simulink library "Actuation_Lib"  (R2026a)
settings: Solver=ode45  EnableMultiTasking=on
undefined symbols (not defined in the file): Mini_Golf_Param, X, Y, Z
libraries: nesl_utility x22, sm_lib x12, Golf_Components_Lib x2, $bdroot x1
Description:
  | Copyright 2015-2026 The MathWorks, Inc.
settings Model: Creator=smiller  LastModifiedBy=smiller
settings DataIOCC: SignalLoggingSaveFormat=ModelDataLogs
settings DebuggingCC: UnderspecifiedInitializationDetection=Classic  PregeneratedLibrarySubsystemCodeDiagnostic=none
settings HardwareCC: ProdHWDeviceType=32-bit Generic

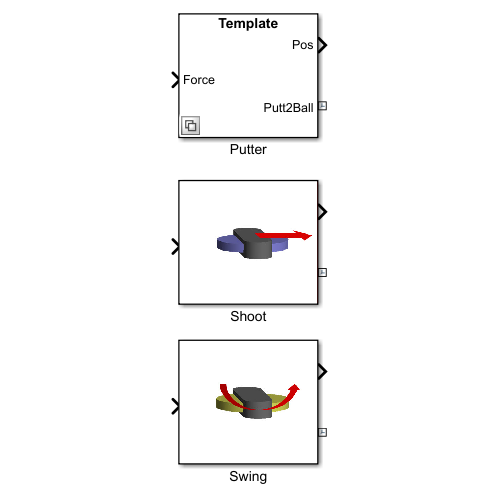
[thumbnail: Simulink's stored preview of the top-level diagram]
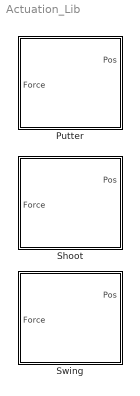
== system Actuation_Lib ==
  Putter : Subsystem  BlockChoice=Shoot
      settings: TemplateBlock=self  MemberBlocks=Shoot,Swing
  Shoot : Subsystem
      mask Display:
      | image(imread('Putter_Shoot_IMAGE.jpg'));
      | %port_label('input',1,'Force');
      | %port_label('output',1,'Pos');
      | %port_label('RConn',1,'Putt2Ball');
  Swing : Subsystem
      mask Display:
      | image(imread('Putter_Swing_IMAGE.jpg'));
      | %port_label('input',1,'Force');
      | %port_label('output',1,'Pos');
      | %port_label('RConn',1,'Putt2Ball');

== system Actuation_Lib/Putter ==
  Force : Inport
  Shoot : $bdroot/Shoot  SystemSampleTime=-1  VariantActivationTime=update diagram  EmptyChoice=off  PassThrough=off  PassThroughVariantControl=(default)  EmptyChoiceVariantControl=(default)  AllowFlexibleInterface=on  Latency=0  AutoFrameSizeCalculation=off
  Putt2Ball : PMIOPort  Side=Right
  Pos : Outport  VectorParamsAs1DForOutWhenUnconnected=off
  wires:
  Force/1 -> Shoot/1
  Shoot/1 -> Pos/1
  connections:
  Shoot/RConn1 -- Putt2Ball/RConn1

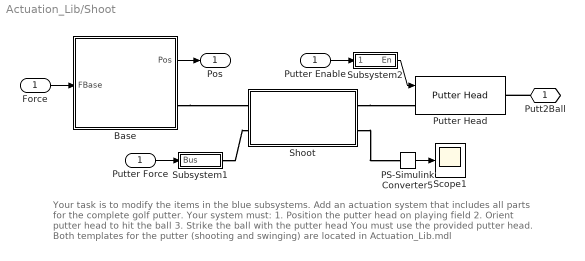
== system Actuation_Lib/Shoot ==
  note: Your task is to modify the items in the blue subsystems.
      | Add an actuation system that includes all parts for the complete golf putter.
      | Your system must:
      | 1. Position the putter head on playing field
      | 2. Orient putter head to hit the ball
      | 3. Strike the ball with the putter head
      |
      | You must use the provided putter head.
      | Both templates for the putter (shooting and swinging) are located in Actuation_Lib.mdl
  Force : Inport
  Base : Subsystem
      mask Display:
      | image(imread('Base_Shoot_IMAGE.jpg'));
      | port_label('input',1,'FBase');
      | port_label('output',1,'Pos');
      | port_label('RConn',1,'CG');
  PS-Simulink Converter5 : nesl_utility/PS-Simulink Converter  PhysicalDomain=network_engine_domain  SubClassName=ps_output  LeftPortType=input  RightPortType=output  PseudoPeriodic=off  Frequencies=[]  VectorFormat=1-D array  Unit=1  AffineConversion=off
  Putter Enable : InportShadow
  Putter Force : InportShadow
  Putter Head : Golf_Components_Lib/Putter Head  length=Mini_Golf_Param.Putter.Length  height=Mini_Golf_Param.Putter.Height  width=Mini_Golf_Param.Putter.Width  ball_radius=Mini_Golf_Param.Ball.Radius  contact_k=Mini_Golf_Param.Wall.Stiffness  contact_b=Mini_Golf_Param.Wall.Damping  low_pass_filt_const=Mini_Golf_Param.Wall.Low_Pass_Filt_Const
  Scope1 : Scope
      settings: DataLoggingVariableName=ScopeData7
  Shoot : Subsystem
      mask Display:
      | image(imread('Shoot_IMAGE.jpg'));
      | port_label('LConn',1,'Actuator');
      | port_label('RConn',1,'Handle');
      | port_label('LConn',2,'Fz');
      | port_label('RConn',2,'p');
  Subsystem1 : Subsystem
  Subsystem2 : Subsystem
  Putt2Ball : PMIOPort  Side=Right
  Pos : Outport  VectorParamsAs1DForOutWhenUnconnected=off
  wires:
  Base/1(Pos) -> Pos/1
  Force/1 -> Base/1(FBase)
  Putter Force/1 -> Subsystem1/1(Bus)
  PS-Simulink Converter5/1 -> Scope1/1
  Putter Enable/1 -> Subsystem2/1(Bus)
  Subsystem2/1(En) -> Putter Head/1
  connections:
  Base/RConn1 -- Shoot/LConn1
  Subsystem1/RConn1 -- Shoot/LConn2
  Shoot/RConn2 -- PS-Simulink Converter5/LConn1
  Putt2Ball/RConn1 -- Putter Head/RConn1
  Shoot/RConn1 -- Putter Head/LConn1

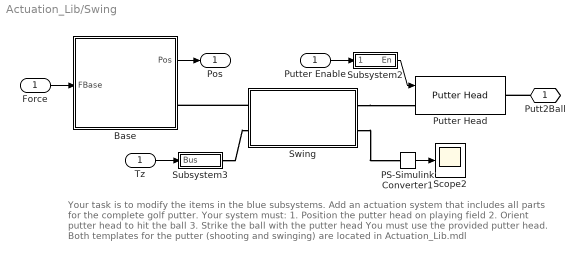
== system Actuation_Lib/Swing ==
  note: Your task is to modify the items in the blue subsystems.
      | Add an actuation system that includes all parts for the complete golf putter.
      | Your system must:
      | 1. Position the putter head on playing field
      | 2. Orient putter head to hit the ball
      | 3. Strike the ball with the putter head
      |
      | You must use the provided putter head.
      | Both templates for the putter (shooting and swinging) are located in Actuation_Lib.mdl
  Force : Inport
  Base : Subsystem
      mask Display:
      | image(imread('Base_Swing_IMAGE.jpg'));
      | port_label('input',1,'FBase');
      | port_label('output',1,'Pos');
      | port_label('RConn',1,'CG');
  PS-Simulink Converter1 : nesl_utility/PS-Simulink Converter  PhysicalDomain=network_engine_domain  SubClassName=ps_output  LeftPortType=input  RightPortType=output  PseudoPeriodic=off  Frequencies=[]  VectorFormat=1-D array  Unit=1  AffineConversion=off
  Putter Enable : InportShadow
  Putter Head : Golf_Components_Lib/Putter Head  length=Mini_Golf_Param.Putter.Length  height=Mini_Golf_Param.Putter.Height  width=Mini_Golf_Param.Putter.Width  ball_radius=Mini_Golf_Param.Ball.Radius  contact_k=Mini_Golf_Param.Wall.Stiffness  contact_b=Mini_Golf_Param.Wall.Damping  low_pass_filt_const=Mini_Golf_Param.Wall.Low_Pass_Filt_Const
  Scope2 : Scope
  Subsystem2 : Subsystem
  Subsystem3 : Subsystem
  Swing : Subsystem
      mask Display:
      | image(imread('Swing_IMAGE.jpg'));
      | port_label('LConn',1,'Actuator');
      | port_label('RConn',1,'Handle');
      | port_label('LConn',2,'Tz');
      | port_label('RConn',2,'p');
  Tz : InportShadow
  Putt2Ball : PMIOPort  Side=Right
  Pos : Outport  VectorParamsAs1DForOutWhenUnconnected=off
  wires:
  Base/1(Pos) -> Pos/1
  Force/1 -> Base/1(FBase)
  Putter Enable/1 -> Subsystem2/1(Bus)
  Subsystem2/1(En) -> Putter Head/1
  Tz/1 -> Subsystem3/1(Bus)
  PS-Simulink Converter1/1 -> Scope2/1
  connections:
  Putt2Ball/RConn1 -- Putter Head/RConn1
  Swing/RConn2 -- PS-Simulink Converter1/LConn1
  Subsystem3/RConn1 -- Swing/LConn2
  Swing/LConn1 -- Base/RConn1
  Swing/RConn1 -- Putter Head/LConn1

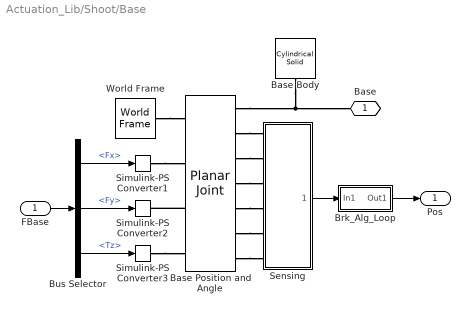
== system Actuation_Lib/Shoot/Base ==
  FBase : Inport
  Base Body : sm_lib/Body Elements/Cylindrical Solid  CylinderRadius=Mini_Golf_Param.Putter.Length*0.5  CylinderRadiusUnits=m  CylinderLength=Mini_Golf_Param.Putter.Height*0.5  CylinderLengthUnits=m  ExportEntireGeometry=off  InertiaType=CalculateFromGeometry  BasedOnType=Mass  Density=1000  DensityUnits=kg/(m^3)  Mass=Mini_Golf_Param.Actuator.Mass  MassUnits=kg  CenterOfMass=[0 0 0]  CenterOfMassUnits=m  MomentsOfInertia=[1 1 1]  MomentsOfInertiaUnits=kg*m^2  ProductsOfInertia=[0 0 0]  ProductsOfInertiaUnits=kg*m^2  GraphicType=FromGeometry  MarkerShape=Sphere  MarkerSize=10  GraphicVisPropType=SimpleVisualProperties  GraphicDiffuseColor=[0.6 0.6 1.0]  GraphicOpacity=1.0  GraphicSpecularColor=[0.5 0.5 0.5 1.0]  GraphicAmbientColor=[0.15 0.15 0.15 1.0]  GraphicEmissiveColor=[0.0 0.0 0.0 1.0]  GraphicShininess=75  DoExposeReferenceFrame=on  SerializedFrames=<Frames/>
  Base Position and Angle : sm_lib/Joints/Planar Joint  JointMode=Normal  CompositeWrenchDir=FollowerOnBase  CompositeWrenchFrame=BaseFrame  SenseConstraintForce=off  SenseConstraintTorque=off  SenseTotalForce=off  SenseTotalTorque=off  PxPositionTargetSpecify=off  PxPositionTargetPriority=High  PxPositionTargetValue=0  PxPositionTargetValueUnits=m  PxVelocityTargetSpecify=off  PxVelocityTargetPriority=High  PxVelocityTargetValue=0  PxVelocityTargetValueUnits=m/s  PxEquilibriumPosition=0  PxEquilibriumPositionUnits=m  PxSpringStiffness=0  PxSpringStiffnessUnits=N/m  PxDampingCoefficient=Mini_Golf_Param.Actuator.Damping_x  PxDampingCoefficientUnits=N/(m/s)  PxLowerLimitSpecify=off  PxLowerLimitBound=-1  PxLowerLimitBoundUnits=m  PxLowerLimitStiffness=1e6  PxLowerLimitStiffnessUnits=N/m  PxLowerLimitDamping=1e3  PxLowerLimitDampingUnits=N/(m/s)  PxLowerLimitTransitionRegionWidth=1e-4  PxLowerLimitTransitionRegionWidthUnits=m  PxUpperLimitSpecify=off  PxUpperLimitBound=1  PxUpperLimitBoundUnits=m  PxUpperLimitStiffness=1e6  PxUpperLimitStiffnessUnits=N/m  PxUpperLimitDamping=1e3  PxUpperLimitDampingUnits=N/(m/s)  PxUpperLimitTransitionRegionWidth=1e-4  PxUpperLimitTransitionRegionWidthUnits=m  PxTorqueActuationMode=InputTorque  PxMotionActuationMode=ComputedMotion  PxSensePosition=on  PxSenseVelocity=on  PxSenseAcceleration=off  PxSenseTorqueForce=off  PxSenseLowerLimitTorqueForce=off  PxSenseUpperLimitTorqueForce=off  PyPositionTargetSpecify=off  PyPositionTargetPriority=High  PyPositionTargetValue=0  PyPositionTargetValueUnits=m  PyVelocityTargetSpecify=off  PyVelocityTargetPriority=High  PyVelocityTargetValue=0  PyVelocityTargetValueUnits=m/s  PyEquilibriumPosition=0  PyEquilibriumPositionUnits=m  PySpringStiffness=0  PySpringStiffnessUnits=N/m  PyDampingCoefficient=Mini_Golf_Param.Actuator.Damping_y  PyDampingCoefficientUnits=N/(m/s)  PyLowerLimitSpecify=off  PyLowerLimitBound=-1  PyLowerLimitBoundUnits=m  PyLowerLimitStiffness=1e6  PyLowerLimitStiffnessUnits=N/m  PyLowerLimitDamping=1e3  PyLowerLimitDampingUnits=N/(m/s)  PyLowerLimitTransitionRegionWidth=1e-4  PyLowerLimitTransitionRegionWidthUnits=m  PyUpperLimitSpecify=off  PyUpperLimitBound=1  PyUpperLimitBoundUnits=m  PyUpperLimitStiffness=1e6  PyUpperLimitStiffnessUnits=N/m  PyUpperLimitDamping=1e3  PyUpperLimitDampingUnits=N/(m/s)  PyUpperLimitTransitionRegionWidth=1e-4  PyUpperLimitTransitionRegionWidthUnits=m  PyTorqueActuationMode=InputTorque  PyMotionActuationMode=ComputedMotion  PySensePosition=on  PySenseVelocity=on  PySenseAcceleration=off  PySenseTorqueForce=off  PySenseLowerLimitTorqueForce=off  PySenseUpperLimitTorqueForce=off  RzPositionTargetSpecify=off  RzPositionTargetPriority=High  RzPositionTargetValue=0  RzPositionTargetValueUnits=rad  RzVelocityTargetSpecify=off  RzVelocityTargetPriority=High  RzVelocityTargetValue=0  RzVelocityTargetValueUnits=rad/s  RzEquilibriumPosition=0  RzEquilibriumPositionUnits=rad  RzSpringStiffness=0  RzSpringStiffnessUnits=N*m/rad  RzDampingCoefficient=Mini_Golf_Param.Actuator.Damping_az  RzDampingCoefficientUnits=N*m/(rad/s)  RzLowerLimitSpecify=off  RzLowerLimitBound=-90  RzLowerLimitBoundUnits=deg  RzLowerLimitStiffness=1e4  RzLowerLimitStiffnessUnits=N*m/deg  RzLowerLimitDamping=10  RzLowerLimitDampingUnits=N*m/(deg/s)  RzLowerLimitTransitionRegionWidth=0.1  RzLowerLimitTransitionRegionWidthUnits=deg  RzUpperLimitSpecify=off  RzUpperLimitBound=90  RzUpperLimitBoundUnits=deg  RzUpperLimitStiffness=1e4  RzUpperLimitStiffnessUnits=N*m/deg  RzUpperLimitDamping=10  RzUpperLimitDampingUnits=N*m/(deg/s)  RzUpperLimitTransitionRegionWidth=0.1  RzUpperLimitTransitionRegionWidthUnits=deg  RzTorqueActuationMode=InputTorque  RzMotionActuationMode=ComputedMotion  RzSensePosition=on  RzSenseVelocity=on  RzSenseAcceleration=off  RzSenseTorqueForce=off  RzSenseLowerLimitTorqueForce=off  RzSenseUpperLimitTorqueForce=off
  Brk_Alg_Loop : Subsystem  mask(First-order lag supporting vector signals){b=Mini_Golf_Param.Actuator.Low_Pass_Filter_Constant, x_initial=0}
      mask prompts: b "Filter time constant"; x_initial "Initial output"
      mask help: Models a lag of the form 1/(b*s+1) where s is the Laplace operator.
  Bus Selector : BusSelector  OutputSignals=Fx,Fy,Tz
  Sensing : Subsystem
  Simulink-PS Converter1 : nesl_utility/Simulink-PS Converter  PhysicalDomain=network_engine_domain  SubClassName=ps_input  LeftPortType=input  RightPortType=output  PseudoPeriodic=off  Frequencies=[]  NoiseDistribution=none  NoiseParameters=[]  Unit=1  AffineConversion=off  FilteringAndDerivatives=zero  SimscapeFilterOrder=1  InputFilterTimeConstant=0.005  UdotUserProvided=0
  Simulink-PS Converter2 : nesl_utility/Simulink-PS Converter  PhysicalDomain=network_engine_domain  SubClassName=ps_input  LeftPortType=input  RightPortType=output  PseudoPeriodic=off  Frequencies=[]  NoiseDistribution=none  NoiseParameters=[]  Unit=1  AffineConversion=off  FilteringAndDerivatives=zero  SimscapeFilterOrder=1  InputFilterTimeConstant=0.005  UdotUserProvided=0
  Simulink-PS Converter3 : nesl_utility/Simulink-PS Converter  PhysicalDomain=network_engine_domain  SubClassName=ps_input  LeftPortType=input  RightPortType=output  PseudoPeriodic=off  Frequencies=[]  NoiseDistribution=none  NoiseParameters=[]  Unit=1  AffineConversion=off  FilteringAndDerivatives=zero  SimscapeFilterOrder=1  InputFilterTimeConstant=0.005  UdotUserProvided=0
  World Frame : sm_lib/Frames and Transforms/World Frame
  Base : PMIOPort  Side=Right
  Pos : Outport  VectorParamsAs1DForOutWhenUnconnected=off
  wires:
  FBase/1 -> Bus Selector/1
  Brk_Alg_Loop/1(Out1) -> Pos/1
  Sensing/1(pos_ang_sig) -> Brk_Alg_Loop/1(In1)
  Bus Selector/1 -> Simulink-PS Converter1/1  "<Fx>"
  Bus Selector/2 -> Simulink-PS Converter2/1  "<Fy>"
  Bus Selector/3 -> Simulink-PS Converter3/1  "<Tz>"
  connections:
  Base Position and Angle/RConn7 -- Sensing/LConn6
  Base Position and Angle/RConn6 -- Sensing/LConn5
  Base Position and Angle/RConn5 -- Sensing/LConn4
  Base Position and Angle/RConn4 -- Sensing/LConn3
  Base Position and Angle/RConn3 -- Sensing/LConn2
  Base Position and Angle/RConn2 -- Sensing/LConn1
  Simulink-PS Converter3/RConn1 -- Base Position and Angle/LConn4
  Base Position and Angle/LConn3 -- Simulink-PS Converter2/RConn1
  Simulink-PS Converter1/RConn1 -- Base Position and Angle/LConn2
  World Frame/RConn1 -- Base Position and Angle/LConn1
  Base Body/RConn1 -- Base Position and Angle/RConn1 -- Base/RConn1

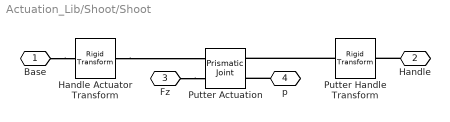
== system Actuation_Lib/Shoot/Shoot ==
  Handle Actuator Transform : sm_lib/Frames and Transforms/Rigid Transform  RotationMethod=StandardAxis  FollAlignAxisA=+X  BaseAlignAxisA=+Y  FollAlignAxisB=+Y  BaseAlignAxisB=+Z  RotationStandardAxis=+Y  RotationAngle=90  RotationAngleUnits=deg  RotationArbitraryAxis=[0 0 1]  RotationSequenceAxes=FollowerAxes  RotationSequence=XYX  RotationSequenceAngles=[0 0 0]  RotationSequenceAnglesUnits=deg  RotationMatrix=[1 0 0; 0 1 0; 0 0 1]  Quaternion=[1 0 0 0]  TranslationMethod=None  TranslationCartesianOffset=[0 0 0]  TranslationCartesianOffsetUnits=m  TranslationStandardAxis=+Z  TranslationStandardOffset=0  TranslationStandardOffsetUnits=m  TranslationROffset=0  TranslationROffsetUnits=m  TranslationThetaOffset=0  TranslationThetaOffsetUnits=deg  TranslationZOffset=0  TranslationZOffsetUnits=m
  Putter Actuation : sm_lib/Joints/Prismatic Joint  JointMode=Normal  CompositeWrenchDir=FollowerOnBase  CompositeWrenchFrame=BaseFrame  SenseConstraintForce=off  SenseConstraintTorque=off  SenseTotalForce=off  SenseTotalTorque=off  PositionTargetSpecify=off  PositionTargetPriority=High  PositionTargetValue=0  PositionTargetValueUnits=m  VelocityTargetSpecify=off  VelocityTargetPriority=High  VelocityTargetValue=0  VelocityTargetValueUnits=m/s  EquilibriumPosition=0  EquilibriumPositionUnits=m  SpringStiffness=Mini_Golf_Param.Actuator.Putter_Spring_k  SpringStiffnessUnits=N/m  DampingCoefficient=Mini_Golf_Param.Actuator.Putter_Damper_b  DampingCoefficientUnits=N/(m/s)  LowerLimitSpecify=off  LowerLimitBound=-1  LowerLimitBoundUnits=m  LowerLimitStiffness=1e6  LowerLimitStiffnessUnits=N/m  LowerLimitDamping=1e3  LowerLimitDampingUnits=N/(m/s)  LowerLimitTransitionRegionWidth=1e-4  LowerLimitTransitionRegionWidthUnits=m  UpperLimitSpecify=off  UpperLimitBound=1  UpperLimitBoundUnits=m  UpperLimitStiffness=1e6  UpperLimitStiffnessUnits=N/m  UpperLimitDamping=1e3  UpperLimitDampingUnits=N/(m/s)  UpperLimitTransitionRegionWidth=1e-4  UpperLimitTransitionRegionWidthUnits=m  TorqueActuationMode=InputTorque  MotionActuationMode=ComputedMotion  SensePosition=on  SenseVelocity=off  SenseAcceleration=off  SenseTorqueForce=off  SenseLowerLimitTorqueForce=off  SenseUpperLimitTorqueForce=off
  Putter Handle Transform : sm_lib/Frames and Transforms/Rigid Transform  RotationMethod=StandardAxis  FollAlignAxisA=+X  BaseAlignAxisA=+Y  FollAlignAxisB=+Y  BaseAlignAxisB=+Z  RotationStandardAxis=+Y  RotationAngle=-90  RotationAngleUnits=deg  RotationArbitraryAxis=[0 0 1]  RotationSequenceAxes=FollowerAxes  RotationSequence=XYX  RotationSequenceAngles=[0 0 0]  RotationSequenceAnglesUnits=deg  RotationMatrix=[1 0 0; 0 1 0; 0 0 1]  Quaternion=[1 0 0 0]  TranslationMethod=None  TranslationCartesianOffset=[0 0 0]  TranslationCartesianOffsetUnits=m  TranslationStandardAxis=+Z  TranslationStandardOffset=0  TranslationStandardOffsetUnits=m  TranslationROffset=0  TranslationROffsetUnits=m  TranslationThetaOffset=0  TranslationThetaOffsetUnits=deg  TranslationZOffset=0  TranslationZOffsetUnits=m
  Base : PMIOPort  Side=Left
  Handle : PMIOPort  Port=2  Side=Right
  Fz : PMIOPort  Port=3  Side=Left
  p : PMIOPort  Port=4  Side=Right
  connections:
  p/RConn1 -- Putter Actuation/RConn2
  Fz/RConn1 -- Putter Actuation/LConn2
  Handle/RConn1 -- Putter Handle Transform/RConn1
  Base/RConn1 -- Handle Actuator Transform/LConn1
  Putter Handle Transform/LConn1 -- Putter Actuation/RConn1
  Handle Actuator Transform/RConn1 -- Putter Actuation/LConn1

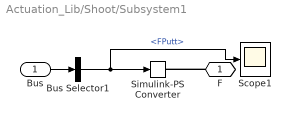
== system Actuation_Lib/Shoot/Subsystem1 ==
  Bus : Inport
  Bus Selector1 : BusSelector  OutputSignals=FPutt
  Scope1 : Scope
      settings: DataLoggingVariableName=ScopeData11
  Simulink-PS Converter : nesl_utility/Simulink-PS Converter  PhysicalDomain=network_engine_domain  SubClassName=ps_input  LeftPortType=input  RightPortType=output  PseudoPeriodic=off  Frequencies=[]  NoiseDistribution=none  NoiseParameters=[]  Unit=1  AffineConversion=off  FilteringAndDerivatives=zero  SimscapeFilterOrder=1  InputFilterTimeConstant=0.005  UdotUserProvided=0
  F : PMIOPort  Side=Right
  wires:
  Bus Selector1/1 -> Simulink-PS Converter/1, Scope1/1  "<FPutt>"
  Bus/1 -> Bus Selector1/1
  connections:
  F/RConn1 -- Simulink-PS Converter/RConn1

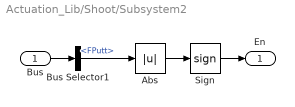
== system Actuation_Lib/Shoot/Subsystem2 ==
  Bus : Inport
  Abs : Abs  SaturateOnIntegerOverflow=off
  Bus Selector1 : BusSelector  OutputSignals=FPutt
  Sign : Signum
  En : Outport  VectorParamsAs1DForOutWhenUnconnected=off
  wires:
  Bus/1 -> Bus Selector1/1
  Abs/1 -> Sign/1
  Bus Selector1/1 -> Abs/1  "<FPutt>"
  Sign/1 -> En/1

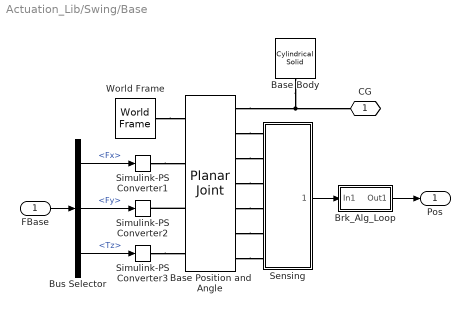
== system Actuation_Lib/Swing/Base ==
  FBase : Inport
  Base Body : sm_lib/Body Elements/Cylindrical Solid  CylinderRadius=Mini_Golf_Param.Putter.Length*0.5  CylinderRadiusUnits=m  CylinderLength=Mini_Golf_Param.Putter.Height*0.5  CylinderLengthUnits=m  ExportEntireGeometry=off  InertiaType=CalculateFromGeometry  BasedOnType=Mass  Density=1000  DensityUnits=kg/(m^3)  Mass=Mini_Golf_Param.Actuator.Mass  MassUnits=kg  CenterOfMass=[0 0 0]  CenterOfMassUnits=m  MomentsOfInertia=[1 1 1]  MomentsOfInertiaUnits=kg*m^2  ProductsOfInertia=[0 0 0]  ProductsOfInertiaUnits=kg*m^2  GraphicType=FromGeometry  MarkerShape=Sphere  MarkerSize=10  GraphicVisPropType=SimpleVisualProperties  GraphicDiffuseColor=[1.0 1.0 0.4]  GraphicOpacity=1.0  GraphicSpecularColor=[0.5 0.5 0.5 1.0]  GraphicAmbientColor=[0.15 0.15 0.15 1.0]  GraphicEmissiveColor=[0.0 0.0 0.0 1.0]  GraphicShininess=75  DoExposeReferenceFrame=on  SerializedFrames=<Frames/>
  Base Position and Angle : sm_lib/Joints/Planar Joint  JointMode=Normal  CompositeWrenchDir=FollowerOnBase  CompositeWrenchFrame=BaseFrame  SenseConstraintForce=off  SenseConstraintTorque=off  SenseTotalForce=off  SenseTotalTorque=off  PxPositionTargetSpecify=off  PxPositionTargetPriority=High  PxPositionTargetValue=0  PxPositionTargetValueUnits=m  PxVelocityTargetSpecify=off  PxVelocityTargetPriority=High  PxVelocityTargetValue=0  PxVelocityTargetValueUnits=m/s  PxEquilibriumPosition=0  PxEquilibriumPositionUnits=m  PxSpringStiffness=0  PxSpringStiffnessUnits=N/m  PxDampingCoefficient=Mini_Golf_Param.Actuator.Damping_x  PxDampingCoefficientUnits=N/(m/s)  PxLowerLimitSpecify=off  PxLowerLimitBound=-1  PxLowerLimitBoundUnits=m  PxLowerLimitStiffness=1e6  PxLowerLimitStiffnessUnits=N/m  PxLowerLimitDamping=1e3  PxLowerLimitDampingUnits=N/(m/s)  PxLowerLimitTransitionRegionWidth=1e-4  PxLowerLimitTransitionRegionWidthUnits=m  PxUpperLimitSpecify=off  PxUpperLimitBound=1  PxUpperLimitBoundUnits=m  PxUpperLimitStiffness=1e6  PxUpperLimitStiffnessUnits=N/m  PxUpperLimitDamping=1e3  PxUpperLimitDampingUnits=N/(m/s)  PxUpperLimitTransitionRegionWidth=1e-4  PxUpperLimitTransitionRegionWidthUnits=m  PxTorqueActuationMode=InputTorque  PxMotionActuationMode=ComputedMotion  PxSensePosition=on  PxSenseVelocity=on  PxSenseAcceleration=off  PxSenseTorqueForce=off  PxSenseLowerLimitTorqueForce=off  PxSenseUpperLimitTorqueForce=off  PyPositionTargetSpecify=off  PyPositionTargetPriority=High  PyPositionTargetValue=0  PyPositionTargetValueUnits=m  PyVelocityTargetSpecify=off  PyVelocityTargetPriority=High  PyVelocityTargetValue=0  PyVelocityTargetValueUnits=m/s  PyEquilibriumPosition=0  PyEquilibriumPositionUnits=m  PySpringStiffness=0  PySpringStiffnessUnits=N/m  PyDampingCoefficient=Mini_Golf_Param.Actuator.Damping_y  PyDampingCoefficientUnits=N/(m/s)  PyLowerLimitSpecify=off  PyLowerLimitBound=-1  PyLowerLimitBoundUnits=m  PyLowerLimitStiffness=1e6  PyLowerLimitStiffnessUnits=N/m  PyLowerLimitDamping=1e3  PyLowerLimitDampingUnits=N/(m/s)  PyLowerLimitTransitionRegionWidth=1e-4  PyLowerLimitTransitionRegionWidthUnits=m  PyUpperLimitSpecify=off  PyUpperLimitBound=1  PyUpperLimitBoundUnits=m  PyUpperLimitStiffness=1e6  PyUpperLimitStiffnessUnits=N/m  PyUpperLimitDamping=1e3  PyUpperLimitDampingUnits=N/(m/s)  PyUpperLimitTransitionRegionWidth=1e-4  PyUpperLimitTransitionRegionWidthUnits=m  PyTorqueActuationMode=InputTorque  PyMotionActuationMode=ComputedMotion  PySensePosition=on  PySenseVelocity=on  PySenseAcceleration=off  PySenseTorqueForce=off  PySenseLowerLimitTorqueForce=off  PySenseUpperLimitTorqueForce=off  RzPositionTargetSpecify=off  RzPositionTargetPriority=High  RzPositionTargetValue=0  RzPositionTargetValueUnits=rad  RzVelocityTargetSpecify=off  RzVelocityTargetPriority=High  RzVelocityTargetValue=0  RzVelocityTargetValueUnits=rad/s  RzEquilibriumPosition=0  RzEquilibriumPositionUnits=rad  RzSpringStiffness=0  RzSpringStiffnessUnits=N*m/rad  RzDampingCoefficient=Mini_Golf_Param.Actuator.Damping_az  RzDampingCoefficientUnits=N*m/(rad/s)  RzLowerLimitSpecify=off  RzLowerLimitBound=-90  RzLowerLimitBoundUnits=deg  RzLowerLimitStiffness=1e4  RzLowerLimitStiffnessUnits=N*m/deg  RzLowerLimitDamping=10  RzLowerLimitDampingUnits=N*m/(deg/s)  RzLowerLimitTransitionRegionWidth=0.1  RzLowerLimitTransitionRegionWidthUnits=deg  RzUpperLimitSpecify=off  RzUpperLimitBound=90  RzUpperLimitBoundUnits=deg  RzUpperLimitStiffness=1e4  RzUpperLimitStiffnessUnits=N*m/deg  RzUpperLimitDamping=10  RzUpperLimitDampingUnits=N*m/(deg/s)  RzUpperLimitTransitionRegionWidth=0.1  RzUpperLimitTransitionRegionWidthUnits=deg  RzTorqueActuationMode=InputTorque  RzMotionActuationMode=ComputedMotion  RzSensePosition=on  RzSenseVelocity=on  RzSenseAcceleration=off  RzSenseTorqueForce=off  RzSenseLowerLimitTorqueForce=off  RzSenseUpperLimitTorqueForce=off
  Brk_Alg_Loop : Subsystem  mask(First-order lag supporting vector signals){b=Mini_Golf_Param.Actuator.Low_Pass_Filter_Constant, x_initial=0}
      mask prompts: b "Filter time constant"; x_initial "Initial output"
      mask help: Models a lag of the form 1/(b*s+1) where s is the Laplace operator.
  Bus Selector : BusSelector  OutputSignals=Fx,Fy,Tz
  Sensing : Subsystem
  Simulink-PS Converter1 : nesl_utility/Simulink-PS Converter  PhysicalDomain=network_engine_domain  SubClassName=ps_input  LeftPortType=input  RightPortType=output  PseudoPeriodic=off  Frequencies=[]  NoiseDistribution=none  NoiseParameters=[]  Unit=1  AffineConversion=off  FilteringAndDerivatives=zero  SimscapeFilterOrder=1  InputFilterTimeConstant=0.005  UdotUserProvided=0
  Simulink-PS Converter2 : nesl_utility/Simulink-PS Converter  PhysicalDomain=network_engine_domain  SubClassName=ps_input  LeftPortType=input  RightPortType=output  PseudoPeriodic=off  Frequencies=[]  NoiseDistribution=none  NoiseParameters=[]  Unit=1  AffineConversion=off  FilteringAndDerivatives=zero  SimscapeFilterOrder=1  InputFilterTimeConstant=0.005  UdotUserProvided=0
  Simulink-PS Converter3 : nesl_utility/Simulink-PS Converter  PhysicalDomain=network_engine_domain  SubClassName=ps_input  LeftPortType=input  RightPortType=output  PseudoPeriodic=off  Frequencies=[]  NoiseDistribution=none  NoiseParameters=[]  Unit=1  AffineConversion=off  FilteringAndDerivatives=zero  SimscapeFilterOrder=1  InputFilterTimeConstant=0.005  UdotUserProvided=0
  World Frame : sm_lib/Frames and Transforms/World Frame
  CG : PMIOPort  Side=Right
  Pos : Outport  VectorParamsAs1DForOutWhenUnconnected=off
  wires:
  FBase/1 -> Bus Selector/1
  Brk_Alg_Loop/1(Out1) -> Pos/1
  Sensing/1(pos_ang_sig) -> Brk_Alg_Loop/1(In1)
  Bus Selector/1 -> Simulink-PS Converter1/1  "<Fx>"
  Bus Selector/2 -> Simulink-PS Converter2/1  "<Fy>"
  Bus Selector/3 -> Simulink-PS Converter3/1  "<Tz>"
  connections:
  Base Position and Angle/RConn7 -- Sensing/LConn6
  Base Position and Angle/RConn6 -- Sensing/LConn5
  Base Position and Angle/RConn5 -- Sensing/LConn4
  Base Position and Angle/RConn4 -- Sensing/LConn3
  Base Position and Angle/RConn3 -- Sensing/LConn2
  Base Position and Angle/RConn2 -- Sensing/LConn1
  Simulink-PS Converter3/RConn1 -- Base Position and Angle/LConn4
  Base Position and Angle/LConn3 -- Simulink-PS Converter2/RConn1
  Simulink-PS Converter1/RConn1 -- Base Position and Angle/LConn2
  World Frame/RConn1 -- Base Position and Angle/LConn1
  Base Body/RConn1 -- Base Position and Angle/RConn1 -- CG/RConn1

== system Actuation_Lib/Swing/Subsystem2 ==
  Bus : Inport
  Abs : Abs  SaturateOnIntegerOverflow=off
  Bus Selector1 : BusSelector  OutputSignals=FPutt
  Sign : Signum
  En : Outport  VectorParamsAs1DForOutWhenUnconnected=off
  wires:
  Bus/1 -> Bus Selector1/1
  Abs/1 -> Sign/1
  Bus Selector1/1 -> Abs/1  "<FPutt>"
  Sign/1 -> En/1

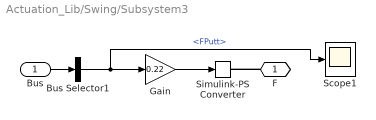
== system Actuation_Lib/Swing/Subsystem3 ==
  Bus : Inport
  Bus Selector1 : BusSelector  OutputSignals=FPutt
  Gain : Gain  Gain=0.22
  Scope1 : Scope
      settings: DataLoggingVariableName=ScopeData11
  Simulink-PS Converter : nesl_utility/Simulink-PS Converter  PhysicalDomain=network_engine_domain  SubClassName=ps_input  LeftPortType=input  RightPortType=output  PseudoPeriodic=off  Frequencies=[]  NoiseDistribution=none  NoiseParameters=[]  Unit=1  AffineConversion=off  FilteringAndDerivatives=zero  SimscapeFilterOrder=1  InputFilterTimeConstant=0.005  UdotUserProvided=0
  F : PMIOPort  Side=Right
  wires:
  Gain/1 -> Simulink-PS Converter/1
  Bus Selector1/1 -> Gain/1, Scope1/1  "<FPutt>"
  Bus/1 -> Bus Selector1/1
  connections:
  F/RConn1 -- Simulink-PS Converter/RConn1

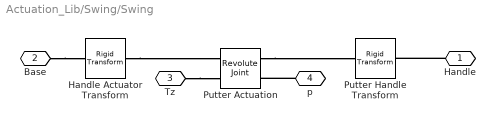
== system Actuation_Lib/Swing/Swing ==
  Handle Actuator Transform : sm_lib/Frames and Transforms/Rigid Transform  RotationMethod=StandardAxis  FollAlignAxisA=+X  BaseAlignAxisA=+Y  FollAlignAxisB=+Y  BaseAlignAxisB=+Z  RotationStandardAxis=+X  RotationAngle=90  RotationAngleUnits=deg  RotationArbitraryAxis=[0 0 1]  RotationSequenceAxes=FollowerAxes  RotationSequence=XYX  RotationSequenceAngles=[0 0 0]  RotationSequenceAnglesUnits=deg  RotationMatrix=[1 0 0; 0 1 0; 0 0 1]  Quaternion=[1 0 0 0]  TranslationMethod=StandardAxis  TranslationCartesianOffset=[0 Mini_Golf_Param.Putter.Length*0.5 0.5]  TranslationCartesianOffsetUnits=m  TranslationStandardAxis=+Z  TranslationStandardOffset=Mini_Golf_Param.Actuator_Swing.Club_Length  TranslationStandardOffsetUnits=m  TranslationROffset=0  TranslationROffsetUnits=m  TranslationThetaOffset=0  TranslationThetaOffsetUnits=deg  TranslationZOffset=0  TranslationZOffsetUnits=m
  Putter Actuation : sm_lib/Joints/Revolute Joint  JointMode=Normal  CompositeWrenchDir=FollowerOnBase  CompositeWrenchFrame=BaseFrame  SenseConstraintForce=off  SenseConstraintTorque=off  SenseTotalForce=off  SenseTotalTorque=off  PositionTargetSpecify=off  PositionTargetPriority=High  PositionTargetValue=0  PositionTargetValueUnits=rad  VelocityTargetSpecify=off  VelocityTargetPriority=High  VelocityTargetValue=0  VelocityTargetValueUnits=rad/s  EquilibriumPosition=0  EquilibriumPositionUnits=rad  SpringStiffness=Mini_Golf_Param.Actuator_Swing.Putter_Spring_k  SpringStiffnessUnits=N*m/rad  DampingCoefficient=Mini_Golf_Param.Actuator_Swing.Putter_Damper_b  DampingCoefficientUnits=N*m/(rad/s)  LowerLimitSpecify=off  LowerLimitBound=-90  LowerLimitBoundUnits=deg  LowerLimitStiffness=1e4  LowerLimitStiffnessUnits=N*m/deg  LowerLimitDamping=10  LowerLimitDampingUnits=N*m/(deg/s)  LowerLimitTransitionRegionWidth=0.1  LowerLimitTransitionRegionWidthUnits=deg  UpperLimitSpecify=off  UpperLimitBound=90  UpperLimitBoundUnits=deg  UpperLimitStiffness=1e4  UpperLimitStiffnessUnits=N*m/deg  UpperLimitDamping=10  UpperLimitDampingUnits=N*m/(deg/s)  UpperLimitTransitionRegionWidth=0.1  UpperLimitTransitionRegionWidthUnits=deg  TorqueActuationMode=InputTorque  MotionActuationMode=ComputedMotion  SensePosition=on  SenseVelocity=off  SenseAcceleration=off  SenseTorqueForce=off  SenseLowerLimitTorqueForce=off  SenseUpperLimitTorqueForce=off
  Putter Handle Transform : sm_lib/Frames and Transforms/Rigid Transform  RotationMethod=StandardAxis  FollAlignAxisA=+X  BaseAlignAxisA=+Y  FollAlignAxisB=+Y  BaseAlignAxisB=+Z  RotationStandardAxis=+X  RotationAngle=-90  RotationAngleUnits=deg  RotationArbitraryAxis=[0 0 1]  RotationSequenceAxes=FollowerAxes  RotationSequence=XYX  RotationSequenceAngles=[0 0 0]  RotationSequenceAnglesUnits=deg  RotationMatrix=[1 0 0; 0 1 0; 0 0 1]  Quaternion=[1 0 0 0]  TranslationMethod=StandardAxis  TranslationCartesianOffset=[0 Mini_Golf_Param.Putter.Length*0.5 0.5]  TranslationCartesianOffsetUnits=m  TranslationStandardAxis=+Y  TranslationStandardOffset=-Mini_Golf_Param.Actuator_Swing.Club_Length  TranslationStandardOffsetUnits=m  TranslationROffset=0  TranslationROffsetUnits=m  TranslationThetaOffset=0  TranslationThetaOffsetUnits=deg  TranslationZOffset=0  TranslationZOffsetUnits=m
  Handle : PMIOPort  Side=Right
  Base : PMIOPort  Port=2  Side=Left
  Tz : PMIOPort  Port=3  Side=Left
  p : PMIOPort  Port=4  Side=Right
  connections:
  Handle Actuator Transform/RConn1 -- Putter Actuation/LConn1
  Putter Actuation/RConn1 -- Putter Handle Transform/LConn1
  Handle/RConn1 -- Putter Handle Transform/RConn1
  Base/RConn1 -- Handle Actuator Transform/LConn1
  Tz/RConn1 -- Putter Actuation/LConn2
  p/RConn1 -- Putter Actuation/RConn2

== system Actuation_Lib/Shoot/Base/Brk_Alg_Loop ==
  In1 : Inport
  Gain : Gain  Gain=1/b
  Integrator : Integrator  InitialCondition=x_initial
  Sum : Sum  Inputs=|+-  InputSameDT=on  SaturateOnIntegerOverflow=on  OutDataTypeStr=Inherit: Same as first input
  Out1 : Outport  VectorParamsAs1DForOutWhenUnconnected=off
  wires:
  Gain/1 -> Out1/1, Sum/2
  Integrator/1 -> Gain/1
  Sum/1 -> Integrator/1
  In1/1 -> Sum/1

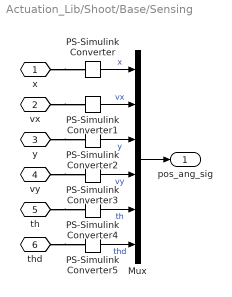
== system Actuation_Lib/Shoot/Base/Sensing ==
  Mux : Mux  Inputs=6
  PS-Simulink Converter{,1..3} (4 alike) : nesl_utility/PS-Simulink Converter  PhysicalDomain=network_engine_domain  SubClassName=ps_output  LeftPortType=input  RightPortType=output  PseudoPeriodic=off  Frequencies=[]  VectorFormat=1-D array  Unit=1  AffineConversion=off
  PS-Simulink Converter4 : nesl_utility/PS-Simulink Converter  PhysicalDomain=network_engine_domain  SubClassName=ps_output  LeftPortType=input  RightPortType=output  PseudoPeriodic=off  Frequencies=[]  VectorFormat=1-D array  Unit=deg  AffineConversion=off
  PS-Simulink Converter5 : nesl_utility/PS-Simulink Converter  PhysicalDomain=network_engine_domain  SubClassName=ps_output  LeftPortType=input  RightPortType=output  PseudoPeriodic=off  Frequencies=[]  VectorFormat=1-D array  Unit=deg/s  AffineConversion=off
  x : PMIOPort  Side=Left
  vx : PMIOPort  Port=2  Side=Left
  y : PMIOPort  Port=3  Side=Left
  vy : PMIOPort  Port=4  Side=Left
  th : PMIOPort  Port=5  Side=Left
  thd : PMIOPort  Port=6  Side=Left
  pos_ang_sig : Outport  VectorParamsAs1DForOutWhenUnconnected=off
  wires:
  PS-Simulink Converter5/1 -> Mux/6  "thd"
  PS-Simulink Converter4/1 -> Mux/5  "th"
  Mux/1 -> pos_ang_sig/1
  PS-Simulink Converter3/1 -> Mux/4  "vy"
  PS-Simulink Converter2/1 -> Mux/3  "y"
  PS-Simulink Converter1/1 -> Mux/2  "vx"
  PS-Simulink Converter/1 -> Mux/1  "x"
  connections:
  thd/RConn1 -- PS-Simulink Converter5/LConn1
  th/RConn1 -- PS-Simulink Converter4/LConn1
  vy/RConn1 -- PS-Simulink Converter3/LConn1
  y/RConn1 -- PS-Simulink Converter2/LConn1
  vx/RConn1 -- PS-Simulink Converter1/LConn1
  x/RConn1 -- PS-Simulink Converter/LConn1

== system Actuation_Lib/Swing/Base/Brk_Alg_Loop ==
  In1 : Inport
  Gain : Gain  Gain=1/b
  Integrator : Integrator  InitialCondition=x_initial
  Sum : Sum  Inputs=|+-  InputSameDT=on  SaturateOnIntegerOverflow=on  OutDataTypeStr=Inherit: Same as first input
  Out1 : Outport  VectorParamsAs1DForOutWhenUnconnected=off
  wires:
  Gain/1 -> Out1/1, Sum/2
  Integrator/1 -> Gain/1
  Sum/1 -> Integrator/1
  In1/1 -> Sum/1

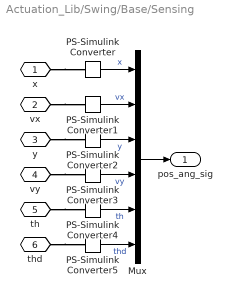
== system Actuation_Lib/Swing/Base/Sensing ==
  Mux : Mux  Inputs=6
  PS-Simulink Converter{,1..3} (4 alike) : nesl_utility/PS-Simulink Converter  PhysicalDomain=network_engine_domain  SubClassName=ps_output  LeftPortType=input  RightPortType=output  PseudoPeriodic=off  Frequencies=[]  VectorFormat=1-D array  Unit=1  AffineConversion=off
  PS-Simulink Converter4 : nesl_utility/PS-Simulink Converter  PhysicalDomain=network_engine_domain  SubClassName=ps_output  LeftPortType=input  RightPortType=output  PseudoPeriodic=off  Frequencies=[]  VectorFormat=1-D array  Unit=deg  AffineConversion=off
  PS-Simulink Converter5 : nesl_utility/PS-Simulink Converter  PhysicalDomain=network_engine_domain  SubClassName=ps_output  LeftPortType=input  RightPortType=output  PseudoPeriodic=off  Frequencies=[]  VectorFormat=1-D array  Unit=deg/s  AffineConversion=off
  x : PMIOPort  Side=Left
  vx : PMIOPort  Port=2  Side=Left
  y : PMIOPort  Port=3  Side=Left
  vy : PMIOPort  Port=4  Side=Left
  th : PMIOPort  Port=5  Side=Left
  thd : PMIOPort  Port=6  Side=Left
  pos_ang_sig : Outport  VectorParamsAs1DForOutWhenUnconnected=off
  wires:
  PS-Simulink Converter5/1 -> Mux/6  "thd"
  PS-Simulink Converter4/1 -> Mux/5  "th"
  Mux/1 -> pos_ang_sig/1
  PS-Simulink Converter3/1 -> Mux/4  "vy"
  PS-Simulink Converter2/1 -> Mux/3  "y"
  PS-Simulink Converter1/1 -> Mux/2  "vx"
  PS-Simulink Converter/1 -> Mux/1  "x"
  connections:
  thd/RConn1 -- PS-Simulink Converter5/LConn1
  th/RConn1 -- PS-Simulink Converter4/LConn1
  vy/RConn1 -- PS-Simulink Converter3/LConn1
  y/RConn1 -- PS-Simulink Converter2/LConn1
  vx/RConn1 -- PS-Simulink Converter1/LConn1
  x/RConn1 -- PS-Simulink Converter/LConn1
